simulink model "modelo_linear"  (R2013a)
settings: Solver=ode45  StartTime=0.0  StopTime=1.5  RelTol=1e-3
values from neighbouring files (symbols this model uses):
  gb = 0.3e-3    (= 0.0003)    [untitled.m]
  gi = 0.7e-3    (= 0.0007)    [untitled.m]
  Kb = E*Hb*Ab/Lb    [untitled.m]
  Kp = 625    [untitled.m]
  L2 = 7.807e-05    [untitled.m]
  m = 0.375    [untitled.m]
  R = 6.3    [untitled.m]
libraries: simulink x2
settings Model: Creator=corsi  LastModifiedBy=rafa
settings OptimizationCC: ExpressionDepthLimit=2147483647

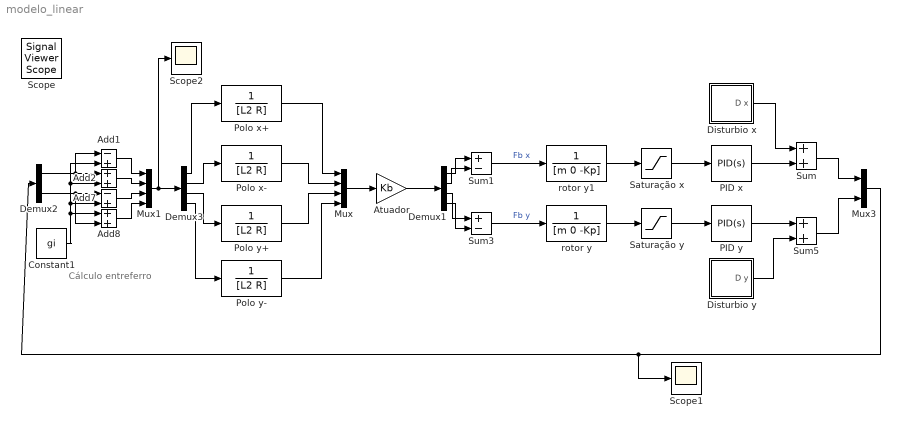
== system modelo_linear ==
  note: Cálculo
      | entreferro
  Add1 : Sum  Inputs=-+
  Add2 : Sum
  Add7 : Sum  Inputs=-+
  Add8 : Sum
  Atuador : Gain  Gain=Kb
  Constant1 : Constant  Value=gi
  Demux1 : Demux
  Demux2 : Demux  Outputs=2
  Demux3 : Demux
  Disturbio x : Subsystem
  Disturbio y : Subsystem
  Mux : Mux
  Mux1 : Mux
  Mux3 : Mux  Inputs=2
  PID x : simulink/Continuous/PID Controller  Controller=PID  TimeDomain=Continuous-time  SampleTime=1  IntegratorMethod=Forward Euler  FilterMethod=Forward Euler  Form=Parallel  P=8.17864953724915  I=11.4602775489375  D=0.0103461841430853  N=5540.04771954153  InitialConditionSource=internal  InitialConditionForIntegrator=0  InitialConditionForFilter=0  ExternalReset=none  LimitOutput=off  UpperSaturationLimit=inf  LowerSaturationLimit=-inf  LinearizeAsGain=on  AntiWindupMode=none  Kb=1  TrackingMode=off  Kt=1  PParamMin=[]  PParamMax=[]  IParamMin=[]  IParamMax=[]  DParamMin=[]  DParamMax=[]  NParamMin=[]  NParamMax=[]  KbParamMin=[]  KbParamMax=[]  KtParamMin=[]  KtParamMax=[]  POutMin=[]  POutMax=[]  IOutMin=[]  IOutMax=[]  DOutMin=[]  DOutMax=[]  NOutMin=[]  NOutMax=[]  KbOutMin=[]  KbOutMax=[]  KtOutMin=[]  KtOutMax=[]  IntegratorOutMin=[]  IntegratorOutMax=[]  FilterOutMin=[]  FilterOutMax=[]  SumOutMin=[]  SumOutMax=[]  SumI1OutMin=[]  SumI1OutMax=[]  SumI2OutMin=[]  SumI2OutMax=[]  SumI3OutMin=[]  SumI3OutMax=[]  SumDOutMin=[]  SumDOutMax=[]  SaturationOutMin=[]  SaturationOutMax=[]  IntegratorContinuousStateAttributes=''  IntegratorStateMustResolveToSignalObject=off  IntegratorRTWStateStorageClass=Auto  FilterContinuousStateAttributes=''  FilterStateMustResolveToSignalObject=off  FilterRTWStateStorageClass=Auto
  PID y : simulink/Continuous/PID Controller  Controller=PID  TimeDomain=Continuous-time  SampleTime=1  IntegratorMethod=Forward Euler  FilterMethod=Forward Euler  Form=Parallel  P=2.58694040908126  I=15.2531990852937  D=0.044459996476507  N=1616.33345877961  InitialConditionSource=internal  InitialConditionForIntegrator=0  InitialConditionForFilter=0  ExternalReset=none  LimitOutput=off  UpperSaturationLimit=inf  LowerSaturationLimit=-inf  LinearizeAsGain=on  AntiWindupMode=none  Kb=1  TrackingMode=off  Kt=1  PParamMin=[]  PParamMax=[]  IParamMin=[]  IParamMax=[]  DParamMin=[]  DParamMax=[]  NParamMin=[]  NParamMax=[]  KbParamMin=[]  KbParamMax=[]  KtParamMin=[]  KtParamMax=[]  POutMin=[]  POutMax=[]  IOutMin=[]  IOutMax=[]  DOutMin=[]  DOutMax=[]  NOutMin=[]  NOutMax=[]  KbOutMin=[]  KbOutMax=[]  KtOutMin=[]  KtOutMax=[]  IntegratorOutMin=[]  IntegratorOutMax=[]  FilterOutMin=[]  FilterOutMax=[]  SumOutMin=[]  SumOutMax=[]  SumI1OutMin=[]  SumI1OutMax=[]  SumI2OutMin=[]  SumI2OutMax=[]  SumI3OutMin=[]  SumI3OutMax=[]  SumDOutMin=[]  SumDOutMax=[]  SaturationOutMin=[]  SaturationOutMax=[]  IntegratorContinuousStateAttributes=''  IntegratorStateMustResolveToSignalObject=off  IntegratorRTWStateStorageClass=Auto  FilterContinuousStateAttributes=''  FilterStateMustResolveToSignalObject=off  FilterRTWStateStorageClass=Auto
  Polo x+ : TransferFcn  Denominator=[L2 R]
  Polo x- : TransferFcn  Denominator=[L2 R]
  Polo y+ : TransferFcn  Denominator=[L2 R]
  Polo y- : TransferFcn  Denominator=[L2 R]
  Saturação x : Saturate  UpperLimit=gb  LowerLimit=-gb
  Saturação y : Saturate  UpperLimit=gb  LowerLimit=-gb
  Scope1 : Scope
      settings: YMin=-5.5e-05  YMax=5.5e-05
  Scope2 : Scope
      settings: YMin=0.000645  YMax=0.000755
  Sum : Sum
  Sum1 : Sum  Inputs=+-
  Sum3 : Sum  Inputs=+-
  Sum5 : Sum
  rotor y : TransferFcn  Denominator=[m 0 -Kp]
  rotor y1 : TransferFcn  Denominator=[m 0 -Kp]
  Scope : SignalViewerScope  IOType=viewer  RefreshTime=0.035000
  wires:
  Polo y+/1 -> Mux/3
  Polo y-/1 -> Mux/4
  Polo x-/1 -> Mux/2
  Polo x+/1 -> Mux/1
  Demux3/1 -> Polo x+/1
  Demux3/2 -> Polo x-/1
  Demux3/3 -> Polo y+/1
  Demux3/4 -> Polo y-/1
  Mux/1 -> Atuador/1
  Demux1/2 -> Sum1/2
  Sum1/1 -> rotor y1/1  "Fb x"
  Demux1/1 -> Sum1/1
  Demux1/3 -> Sum3/1
  Atuador/1 -> Demux1/1
  Demux1/4 -> Sum3/2
  Demux2/2 -> Add8/2, Add7/1
  Constant1/1 -> Add2/2, Add1/2, Add7/2, Add8/1
  Demux2/1 -> Add1/1, Add2/1
  Add1/1 -> Mux1/1
  Add2/1 -> Mux1/2
  Add7/1 -> Mux1/3
  Add8/1 -> Mux1/4
  Mux1/1 -> Scope2/1, Demux3/1
  Saturação x/1 -> PID x/1
  Sum3/1 -> rotor y/1  "Fb y"
  rotor y/1 -> Saturação y/1
  rotor y1/1 -> Saturação x/1
  Saturação y/1 -> PID y/1
  Mux3/1 -> Scope1/1, Demux2/1
  Disturbio x/1(D x) -> Sum/1
  PID x/1 -> Sum/2
  PID y/1 -> Sum5/1
  Sum/1 -> Mux3/1
  Sum5/1 -> Mux3/2
  Disturbio y/1(D y) -> Sum5/2

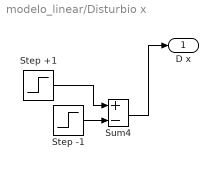
== system modelo_linear/Disturbio x ==
  Step +1 : Step  Time=0.8  After=0.05E-3
  Step -1 : Step  Time=0.15  After=0.05E-3
  Sum4 : Sum  Inputs=+-
  D x : Outport
  wires:
  Step +1/1 -> Sum4/1
  Step -1/1 -> Sum4/2
  Sum4/1 -> D x/1

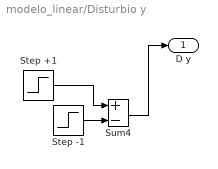
== system modelo_linear/Disturbio y ==
  Step +1 : Step  Time=0.3  After=0.05E-3
  Step -1 : Step  Time=0.5  After=0.05E-3
  Sum4 : Sum  Inputs=+-
  D y : Outport
  wires:
  Step +1/1 -> Sum4/1
  Step -1/1 -> Sum4/2
  Sum4/1 -> D y/1
